simulink model "Transmission_Library"  (Simulink 7.6)
settings: Solver=ode45  StartTime=0.0  StopTime=10.0  RelTol=1e-3
PostLoadFcn:
  | %%% BEGIN TransmissionOne CODE %%%
  | % Import the data from Excel for a lookup table
  | data = xlsread('Transmission_Specification.xlsx', 'TransmissionOne');
  | for idx=1:length(data(:,1))
  | if isnan(data(idx,1))
  |   break
  | end
  | Transmission_TransmissionOne_FWD_gear_number_raw(idx) = data(idx,1);
  | end
  | for idx=1:length(data(:,2))
  | if isnan(data(idx,2))
  |   break
  | end
  | Transmission_TransmissionOne_FWD_gear_ratio_raw(idx) = data(idx,2);
  | end
  | if length(Transmission_TransmissionOne_FWD_gear_ratio_raw) ~= length(Transmission_TransmissionOne_FWD_gear_number_raw)
  | disp('ERROR: TransmissionOne_FWD_gear_number and TransmissionOne_FWD_gear_ratio sizes are not match. Fix it in excel.');
  | end
  | for idx=1:length(data(:,3))
  | if isnan(data(idx,3))
  |   break
  | end
  | Transmission_TransmissionOne_Reverse_gear_ratio_raw(idx) = data(idx,3);
  | end
  | for idx=1:length(data(:,4))
  | if isnan(data(idx,4))
  |   break
  | end
  | Transmission_TransmissionOne_Reverse_gear_number_raw(idx) = data(idx,4);
  | end
  | if length(Transmission_TransmissionOne_Reverse_gear_ratio_raw) ~= length(Transmission_TransmissionOne_Reverse_gear_number_raw)
  | disp('ERROR: TransmissionOne_Reverse_gear_number and TransmissionOne_Reverse_gear_ratio sizes are not match. Fix it in excel.');
  | end
  | %%% END TransmissionOne CODE %%%%%% BEGIN TransmissionTwo CODE %%%
  | % Import the data from Excel for a lookup table
  | data = xlsread('Transmission_Specification.xlsx', 'TransmissionTwo');
  | for idx=1:length(data(:,1))
  | if isnan(data(idx,1))
  |   break
  | end
  | Transmission_TransmissionTwo_FWD_gear_number_raw(idx) = data(idx,1);
  | end
  | for idx=1:length(data(:,2))
  | if isnan(data(idx,2))
  |   break
  | end
  | Transmission_TransmissionTwo_FWD_gear_ratio_raw(idx) = data(idx,2);
  | end
  | if length(Transmission_TransmissionTwo_FWD_gear_ratio_raw) ~= length(Transmission_TransmissionTwo_FWD_gear_number_raw)
  | disp('ERROR: TransmissionTwo_FWD_gear_number and TransmissionTwo_FWD_gear_ratio sizes are not match. Fix it in excel.');
  | end
  | for idx=1:length(data(:,3))
  | if isnan(data(idx,3))
  |   break
  | end
  | Transmission_TransmissionTwo_Reverse_gear_ratio_raw(idx) = data(idx,3);
  | end
  | for idx=1:length(data(:,4))
  | if isnan(data(idx,4))
  |   break
  | end
  | Transmission_TransmissionTwo_Reverse_gear_number_raw(idx) = data(idx,4);
  | end
  | if length(Transmission_TransmissionTwo_Reverse_gear_ratio_raw) ~= length(Transmission_TransmissionTwo_Reverse_gear_number_raw)
  | disp('ERROR: TransmissionTwo_Reverse_gear_number and TransmissionTwo_Reverse_gear_ratio sizes are not match. Fix it in excel.');
  | end
  | %%% END TransmissionTwo CODE %%%%%% BEGIN TransmissionThree CODE %%%
  | % Import the data from Excel for a lookup table
  | data = xlsread('Transmission_Specification.xlsx', 'TransmissionThree');
  | for idx=1:length(data(:,1))
  | if isnan(data(idx,1))
  |   break
  | end
  | Transmission_TransmissionThree_FWD_gear_number_raw(idx) = data(idx,1);
  | end
  | for idx=1:length(data(:,2))
  | if isnan(data(idx,2))
  |   break
  | end
  | Transmission_TransmissionThree_FWD_gear_ratio_raw(idx) = data(idx,2);
  | end
  | if length(Transmission_TransmissionThree_FWD_gear_ratio_raw) ~= length(Transmission_TransmissionThree_FWD_gear_number_raw)
  | disp('ERROR: TransmissionThree_FWD_gear_number and TransmissionThree_FWD_gear_ratio sizes are not match. Fix it in excel.');
  | end
  | for idx=1:length(data(:,3))
  | if isnan(data(idx,3))
  |   break
  | end
  | Transmission_TransmissionThree_Reverse_gear_ratio_raw(idx) = data(idx,3);
  | end
  | for idx=1:length(data(:,4))
  | if isnan(data(idx,4))
  |   break
  | end
  | Transmission_TransmissionThree_Reverse_gear_number_raw(idx) = data(idx,4);
  | end
  | if length(Transmission_TransmissionThree_Reverse_gear_ratio_raw) ~= length(Transmission_TransmissionThree_Reverse_gear_number_raw)
  | disp('ERROR: TransmissionThree_Reverse_gear_number and TransmissionThree_Reverse_gear_ratio sizes are not match. Fix it in excel.');
  | end
  | %%% END TransmissionThree CODE %%%
undefined symbols (not defined in the file): Transmission_TransmissionOne_FWD_gear_number_raw, Transmission_TransmissionOne_FWD_gear_ratio_raw, Transmission_TransmissionOne_Reverse_gear_number_raw, Transmission_TransmissionOne_Reverse_gear_ratio_raw, Transmission_TransmissionThree_FWD_gear_number_raw, Transmission_TransmissionThree_FWD_gear_ratio_raw, Transmission_TransmissionThree_Reverse_gear_number_raw, Transmission_TransmissionThree_Reverse_gear_ratio_raw, Transmission_TransmissionTwo_FWD_gear_number_raw, Transmission_TransmissionTwo_FWD_gear_ratio_raw, Transmission_TransmissionTwo_Reverse_gear_number_raw, Transmission_TransmissionTwo_Reverse_gear_ratio_raw
settings Model: Creator=Zsolt  LastModifiedBy=Zsolt
settings HardwareCC: TargetIntDivRoundTo=Zero  TargetEndianess=LittleEndian  TargetHWDeviceType=MATLAB Host  ProdEqTarget=off
settings RTWCC: SystemTargetFile=rsim.tlc  TemplateMakefile=rsim_default_tmf  Description=Rapid Simulation Target  ProcessScript=rsim_make_rtw_hook
settings RSimTargetCC: TargetFunctionLibrary=ANSI_C  ERTMultiwordTypeDef=System defined  ERTCodeCoverageTool=None  ERTMultiwordLength=256  IsPILTarget=off  EnableShiftOperators=on  PortableWordSizes=off

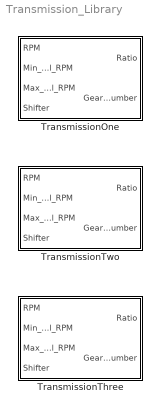
== system Transmission_Library ==
  TransmissionOne : Subsystem
  TransmissionThree : Subsystem
  TransmissionTwo : Subsystem

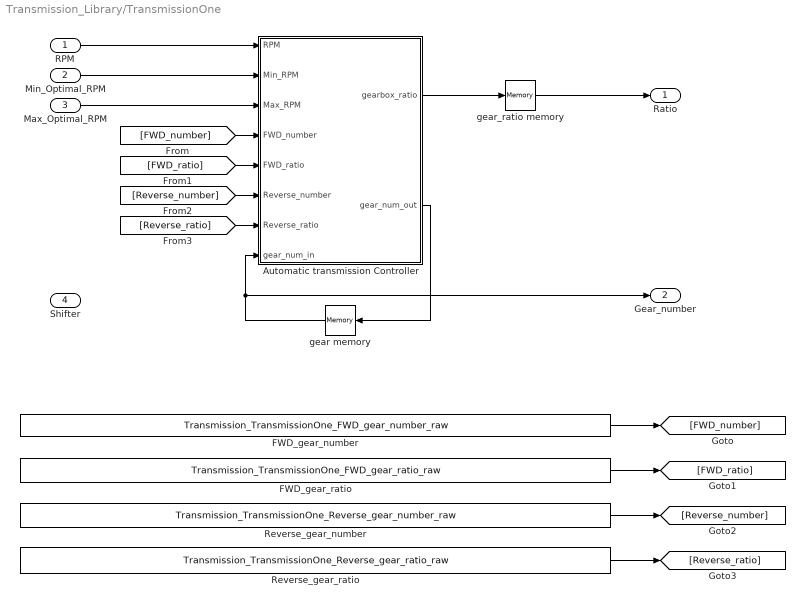
== system Transmission_Library/TransmissionOne ==
  RPM : Inport
  Min_Optimal_RPM : Inport  Port=2
  Max_Optimal_RPM : Inport  Port=3
  Shifter : Inport  Port=4
  Automatic transmission Controller : Stateflow chart  TreatAsAtomicUnit=on
  FWD_gear_number : Constant  Value=Transmission_TransmissionOne_FWD_gear_number_raw
  FWD_gear_ratio : Constant  Value=Transmission_TransmissionOne_FWD_gear_ratio_raw
  Reverse_gear_number : Constant  Value=Transmission_TransmissionOne_Reverse_gear_number_raw
  Reverse_gear_ratio : Constant  Value=Transmission_TransmissionOne_Reverse_gear_ratio_raw
  gear memory : Memory  X0=1
  gear_ratio memory : Memory  X0=1
  Ratio : Outport
  Gear_number : Outport  Port=2
  wires:
  [Reverse_ratio] -> Automatic transmission Controller/7(Reverse_ratio)
  [Reverse_number] -> Automatic transmission Controller/6(Reverse_number)
  [FWD_ratio] -> Automatic transmission Controller/5(FWD_ratio)
  [FWD_number] -> Automatic transmission Controller/4(FWD_number)
  Max_Optimal_RPM/1 -> Automatic transmission Controller/3(Max_RPM)
  Min_Optimal_RPM/1 -> Automatic transmission Controller/2(Min_RPM)
  RPM/1 -> Automatic transmission Controller/1(RPM)
  gear_ratio memory/1 -> Ratio/1
  Automatic transmission Controller/1(gearbox_ratio) -> gear_ratio memory/1
  Automatic transmission Controller/2(gear_num_out) -> gear memory/1
  gear memory/1 -> Gear_number/1, Automatic transmission Controller/8(gear_num_in)
  Reverse_gear_ratio/1 -> [Reverse_ratio]
  Reverse_gear_number/1 -> [Reverse_number]
  FWD_gear_ratio/1 -> [FWD_ratio]
  FWD_gear_number/1 -> [FWD_number]

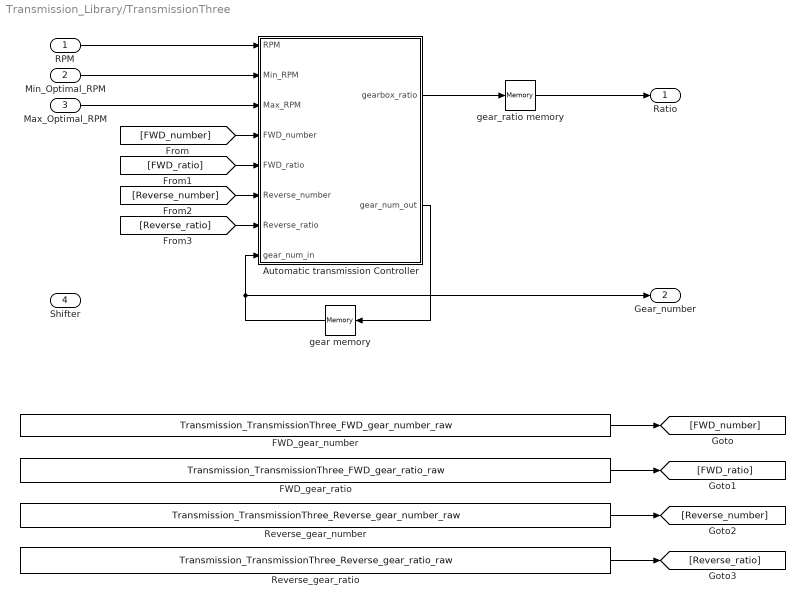
== system Transmission_Library/TransmissionThree ==
  RPM : Inport
  Min_Optimal_RPM : Inport  Port=2
  Max_Optimal_RPM : Inport  Port=3
  Shifter : Inport  Port=4
  Automatic transmission Controller : Stateflow chart  TreatAsAtomicUnit=on
  FWD_gear_number : Constant  Value=Transmission_TransmissionThree_FWD_gear_number_raw
  FWD_gear_ratio : Constant  Value=Transmission_TransmissionThree_FWD_gear_ratio_raw
  Reverse_gear_number : Constant  Value=Transmission_TransmissionThree_Reverse_gear_number_raw
  Reverse_gear_ratio : Constant  Value=Transmission_TransmissionThree_Reverse_gear_ratio_raw
  gear memory : Memory  X0=1
  gear_ratio memory : Memory  X0=1
  Ratio : Outport
  Gear_number : Outport  Port=2
  wires:
  [Reverse_ratio] -> Automatic transmission Controller/7(Reverse_ratio)
  [Reverse_number] -> Automatic transmission Controller/6(Reverse_number)
  [FWD_ratio] -> Automatic transmission Controller/5(FWD_ratio)
  [FWD_number] -> Automatic transmission Controller/4(FWD_number)
  Max_Optimal_RPM/1 -> Automatic transmission Controller/3(Max_RPM)
  Min_Optimal_RPM/1 -> Automatic transmission Controller/2(Min_RPM)
  RPM/1 -> Automatic transmission Controller/1(RPM)
  gear_ratio memory/1 -> Ratio/1
  Automatic transmission Controller/1(gearbox_ratio) -> gear_ratio memory/1
  Automatic transmission Controller/2(gear_num_out) -> gear memory/1
  gear memory/1 -> Gear_number/1, Automatic transmission Controller/8(gear_num_in)
  Reverse_gear_ratio/1 -> [Reverse_ratio]
  Reverse_gear_number/1 -> [Reverse_number]
  FWD_gear_ratio/1 -> [FWD_ratio]
  FWD_gear_number/1 -> [FWD_number]

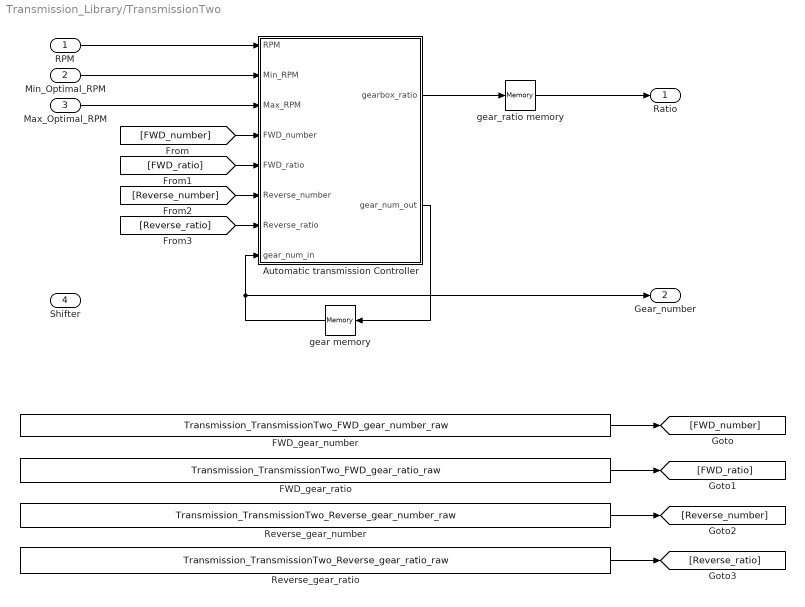
== system Transmission_Library/TransmissionTwo ==
  RPM : Inport
  Min_Optimal_RPM : Inport  Port=2
  Max_Optimal_RPM : Inport  Port=3
  Shifter : Inport  Port=4
  Automatic transmission Controller : Stateflow chart  TreatAsAtomicUnit=on
  FWD_gear_number : Constant  Value=Transmission_TransmissionTwo_FWD_gear_number_raw
  FWD_gear_ratio : Constant  Value=Transmission_TransmissionTwo_FWD_gear_ratio_raw
  Reverse_gear_number : Constant  Value=Transmission_TransmissionTwo_Reverse_gear_number_raw
  Reverse_gear_ratio : Constant  Value=Transmission_TransmissionTwo_Reverse_gear_ratio_raw
  gear memory : Memory  X0=1
  gear_ratio memory : Memory  X0=1
  Ratio : Outport
  Gear_number : Outport  Port=2
  wires:
  [Reverse_ratio] -> Automatic transmission Controller/7(Reverse_ratio)
  [Reverse_number] -> Automatic transmission Controller/6(Reverse_number)
  [FWD_ratio] -> Automatic transmission Controller/5(FWD_ratio)
  [FWD_number] -> Automatic transmission Controller/4(FWD_number)
  Max_Optimal_RPM/1 -> Automatic transmission Controller/3(Max_RPM)
  Min_Optimal_RPM/1 -> Automatic transmission Controller/2(Min_RPM)
  RPM/1 -> Automatic transmission Controller/1(RPM)
  gear_ratio memory/1 -> Ratio/1
  Automatic transmission Controller/1(gearbox_ratio) -> gear_ratio memory/1
  Automatic transmission Controller/2(gear_num_out) -> gear memory/1
  gear memory/1 -> Gear_number/1, Automatic transmission Controller/8(gear_num_in)
  Reverse_gear_ratio/1 -> [Reverse_ratio]
  Reverse_gear_number/1 -> [Reverse_number]
  FWD_gear_ratio/1 -> [FWD_ratio]
  FWD_gear_number/1 -> [FWD_number]

== matlab function TransmissionTwo/Automatic transmission Controller ==
  data: gearbox_ratio output double; RPM input double; Min_RPM input double; Max_RPM input double; FWD_number input double; FWD_ratio input double; Reverse_number input double; Reverse_ratio input double; gear_num_out output double; gear_num_in input double
function [gearbox_ratio, gear_num_out] = fcn(RPM, ...
                                             Min_RPM, ...
                                             Max_RPM, ...
                                             FWD_number, ...
                                             FWD_ratio, ...
                                             Reverse_number, ...
                                             Reverse_ratio, ...
                                             gear_num_in)
%#eml

gear_num_out = gear_num_in;
%gearbox_ratio = 0.12/min(FWD_number);


if (RPM > Max_RPM) && (gear_num_in < max(FWD_number))
    gear_num_out = gear_num_in + 1;    
elseif (RPM < Min_RPM) && (gear_num_in > min(FWD_number))
    gear_num_out = gear_num_in - 1;
end

r = find(FWD_number == gear_num_out);
rr = FWD_ratio(r(1));
gearbox_ratio = rr(1);
% gearbox_ratio = FWD_ratio(find(FWD_number == gear_num_out));

% switch gear_num_out
%     case 1
%         gearbox_ratio = 0.12/3.5;
%     case 2
%         gearbox_ratio = 0.12/2.2;        
%     case 3
%         gearbox_ratio = 0.12/1.4;        
%     case 4
%         gearbox_ratio = 0.12/1;
end

== matlab function TransmissionThree/Automatic transmission Controller ==
  data: gearbox_ratio output double; RPM input double; Min_RPM input double; Max_RPM input double; FWD_number input double; FWD_ratio input double; Reverse_number input double; Reverse_ratio input double; gear_num_out output double; gear_num_in input double
function [gearbox_ratio, gear_num_out] = fcn(RPM, ...
                                             Min_RPM, ...
                                             Max_RPM, ...
                                             FWD_number, ...
                                             FWD_ratio, ...
                                             Reverse_number, ...
                                             Reverse_ratio, ...
                                             gear_num_in)
%#eml

gear_num_out = gear_num_in;
%gearbox_ratio = 0.12/min(FWD_number);


if (RPM > Max_RPM) && (gear_num_in < max(FWD_number))
    gear_num_out = gear_num_in + 1;    
elseif (RPM < Min_RPM) && (gear_num_in > min(FWD_number))
    gear_num_out = gear_num_in - 1;
end

r = find(FWD_number == gear_num_out);
rr = FWD_ratio(r(1));
gearbox_ratio = rr(1);
% gearbox_ratio = FWD_ratio(find(FWD_number == gear_num_out));

% switch gear_num_out
%     case 1
%         gearbox_ratio = 0.12/3.5;
%     case 2
%         gearbox_ratio = 0.12/2.2;        
%     case 3
%         gearbox_ratio = 0.12/1.4;        
%     case 4
%         gearbox_ratio = 0.12/1;
end

== matlab function TransmissionOne/Automatic transmission Controller ==
  data: gearbox_ratio output double; RPM input double; Min_RPM input double; Max_RPM input double; FWD_number input double; FWD_ratio input double; Reverse_number input double; Reverse_ratio input double; gear_num_out output double; gear_num_in input double
function [gearbox_ratio, gear_num_out] = fcn(RPM, ...
                                             Min_RPM, ...
                                             Max_RPM, ...
                                             FWD_number, ...
                                             FWD_ratio, ...
                                             Reverse_number, ...
                                             Reverse_ratio, ...
                                             gear_num_in)
%#eml

gear_num_out = gear_num_in;
%gearbox_ratio = 0.12/min(FWD_number);


if (RPM > Max_RPM) && (gear_num_in < max(FWD_number))
    gear_num_out = gear_num_in + 1;    
elseif (RPM < Min_RPM) && (gear_num_in > min(FWD_number))
    gear_num_out = gear_num_in - 1;
end

r = find(FWD_number == gear_num_out);
rr = FWD_ratio(r(1));
gearbox_ratio = rr(1);
% gearbox_ratio = FWD_ratio(find(FWD_number == gear_num_out));

% switch gear_num_out
%     case 1
%         gearbox_ratio = 0.12/3.5;
%     case 2
%         gearbox_ratio = 0.12/2.2;        
%     case 3
%         gearbox_ratio = 0.12/1.4;        
%     case 4
%         gearbox_ratio = 0.12/1;
end
